simulink model "threephases"  (R2013a)
settings: Solver=ode45  StartTime=0.0  StopTime=1.0  RelTol=1e-3
libraries: powerlib x9, electricdrivelib x1, fl_lib x1
settings Model: Creator=hp  LastModifiedBy=hp

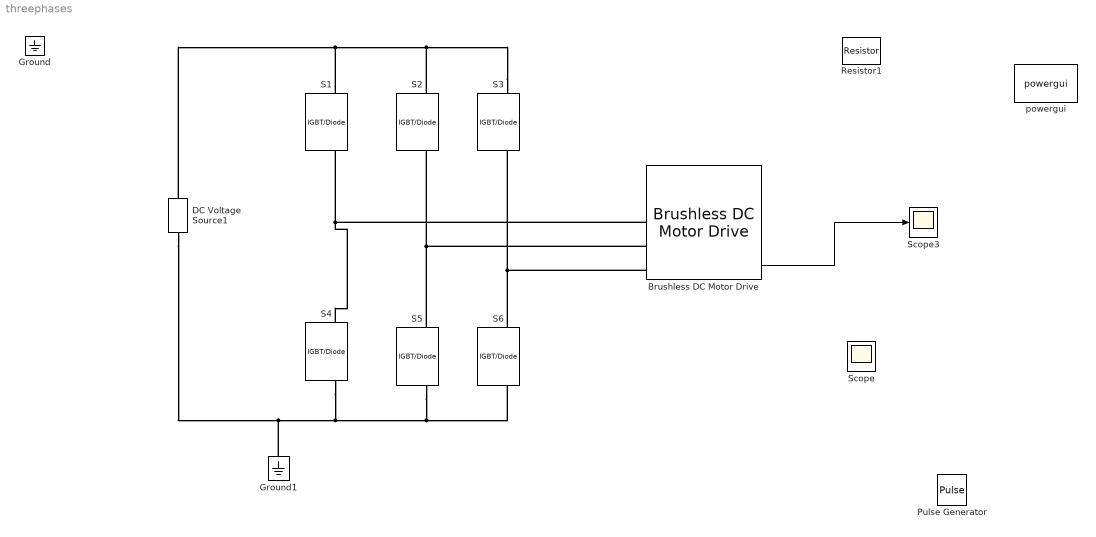
== system threephases ==
  Brushless DC Motor Drive : electricdrivelib/AC drives/Brushless DC Motor Drive  showMaskWarnings=on  AverageValue=off  MechanicalLoad=Torque Tm  driveType=AC7
  DC Voltage Source1 : powerlib/Electrical Sources/DC Voltage Source  Amplitude=240  Measurements=None
  Ground : Ground
  Ground1 : powerlib/Elements/Ground  LConnTagsString=a
  Pulse Generator : DiscretePulseGenerator  PulseType=Time based  Period=10  PulseWidth=5
  Resistor1 : fl_lib/Electrical/Electrical Elements/Resistor  R=1 Ohm  i_Log=off  v_Log=off  LocalVarNames=|i|v  LocalVarDescs=|i|v  LocalVarLogging=[0 0]
  S{1..6} (6 alike) : powerlib/Power Electronics/IGBT//Diode  Ron=1e-3  Rs=1e5  Cs=inf  Measurements=on
  Scope : Scope
      settings: Floating=on
  Scope3 : Scope
      settings: SaveName=IC
  powergui : powerlib/powergui  Priority=1  SimulationMode=Discrete  SolverType=Tustin  SampleTime=1e-6  frequency=60  SPID=off  DisableSnubberDevices=off  DisableRonSwitches=off  DisableVfSwitches=off  SwTol=0  Interpol=off  DisplayEquations=off  frequencyindice=0  Pbase=100e6  ErrMax=1e-4  Iterations=50  UnitsV=kV  UnitsW=MW  FunctionMessages=off  echomessages=off  HookPort=off  EnableUseOfTLC=off  x0status=blocks  RestoreLinks=warning  ResistiveCurrentMeasurement=off  Frange=[0:2:500]  Ylog=off  Xlog=on  ShowGrid=off  save=off  variable=ZData  ZoomFFT=off  StartTime=0.0  cycles=1  DisplayStyle=1  fundamental=60  FreqAxis=off  MaxFrequency=1000  frequencyindicesteady=1  RmsSteady=1  display=off  Ts=0  methode=off
  wires:
  Brushless DC Motor Drive/4 -> Scope3/1
  connections:
  S6/LConn1 -- Brushless DC Motor Drive/LConn3 -- S3/RConn1
  S4/RConn1 -- Ground1/LConn1 -- DC Voltage Source1/LConn1 -- S5/RConn1 -- S6/RConn1
  S3/LConn1 -- S2/LConn1 -- DC Voltage Source1/RConn1 -- S1/LConn1
  S4/LConn1 -- Brushless DC Motor Drive/LConn1 -- S1/RConn1
  S5/LConn1 -- Brushless DC Motor Drive/LConn2 -- S2/RConn1
